simulink model "model_func"  (R2024b)
settings: Solver=VariableStepAuto  StartTime=0.0  StopTime=10.0  RelTol=1e-3
settings Model: Creator=gabrijela  LastModifiedBy=gabrijela

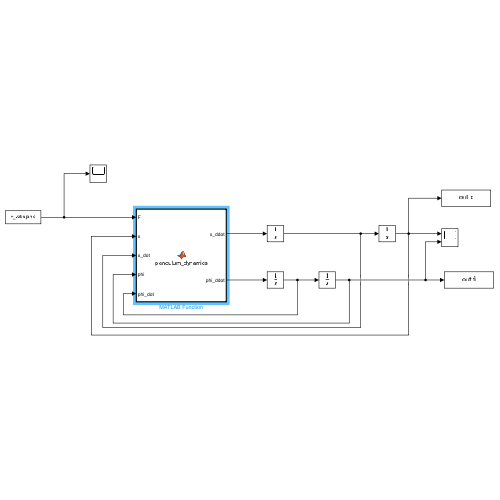
[thumbnail: Simulink's stored preview of the top-level diagram]
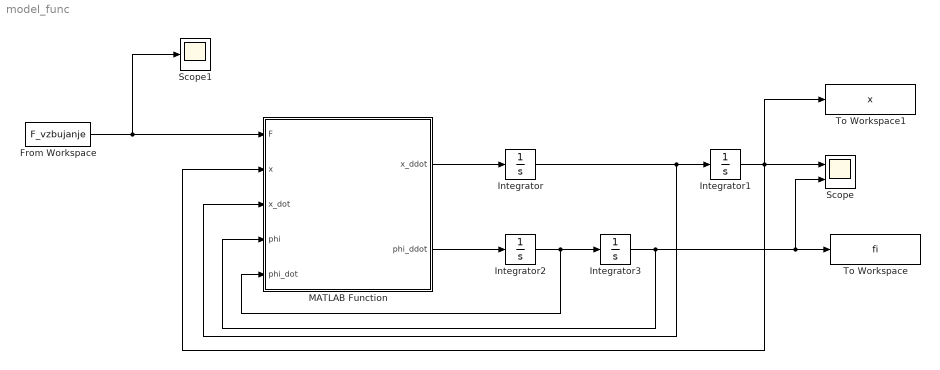
== system model_func ==
  From Workspace : FromWorkspace  VariableName=F_vzbujanje
  Integrator{,1..3} (4 alike) : Integrator
  MATLAB Function : MATLAB Function  TreatAsAtomicUnit=on
  Scope : Scope  NumInputPorts=2
  Scope1 : Scope
  To Workspace : ToWorkspace  VariableName=fi  SaveFormat=Timeseries  SampleTime=-1
  To Workspace1 : ToWorkspace  VariableName=x  SaveFormat=Timeseries  SampleTime=-1
  wires:
  MATLAB Function/2(phi_ddot) -> Integrator2/1
  MATLAB Function/1(x_ddot) -> Integrator/1
  Integrator2/1 -> MATLAB Function/5(phi_dot), Integrator3/1
  Integrator/1 -> MATLAB Function/3(x_dot), Integrator1/1
  Integrator1/1 -> To Workspace1/1, Scope/1, MATLAB Function/2(x)
  From Workspace/1 -> Scope1/1, MATLAB Function/1(F)
  Integrator3/1 -> MATLAB Function/4(phi), To Workspace/1, Scope/2

== matlab function model_func/MATLAB Function ==
  data: F input; x_ddot output; x input; x_dot input; phi input; phi_dot input; phi_ddot output
function [x_ddot, phi_ddot] = pendulum_dynamics(F, x, x_dot, phi, phi_dot)
    % Define parameters
    m1 = 2;           % Mass of the cart (kg)
    m2 = 0.31;        % Mass of the pendulum (kg)
    l = 0.5;          % Length of the pendulum (m)
    f1 = 10;          % Damping constant for the cart (kg/s)
    f2 = 0.00145;     % Damping constant for the pendulum (kg·m^2/s)
    J = 0.08433;      % Pendulum inertia (kg·m^2)
    g = 9.81;         % Gravitational acceleration (m/s^2)

    % Precompute constants
    c1 = 1 / (m1 + m2);
    c2 = 1 / (J + (m2^2 * l^2) / (m1 + m2));

    % Compute cart acceleration (x_ddot)
    x_ddot = c1 * (F - f1 * x_dot + (m2 * l / J) * (f2 * phi_dot + m2 * l * g * phi));

    % Compute pendulum angular acceleration (phi_ddot)
    phi_ddot = -c2 * (f2 * phi_dot + m2 * l * g * phi - (m2 * l / (m1 + m2)) * F + ...
                      (m2 * l * f1 / (m1 + m2)) * x_dot);
end
